simulink model "LinksMotorLinksAbbiegen"  (R2012b)
settings: Solver=ode45  StartTime=0.0  StopTime=11.0  RelTol=1e-3
undefined symbols (not defined in the file): sigbuilder_block
settings Model: Creator=mit064  LastModifiedBy=mit064

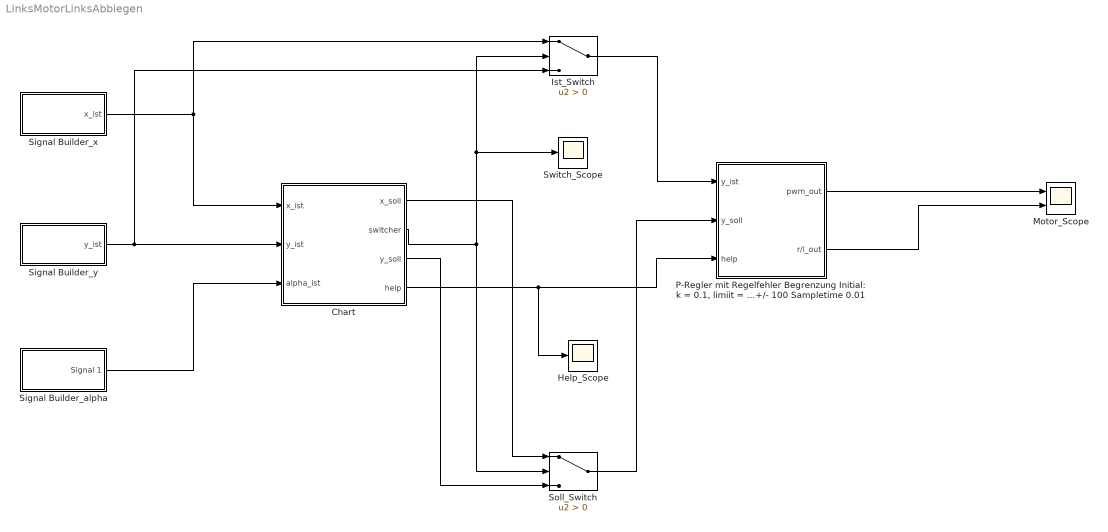
== system LinksMotorLinksAbbiegen ==
  Chart : Stateflow chart  TreatAsAtomicUnit=on
  Help_Scope : Scope
  Ist_Switch : Switch  Criteria=u2 > Threshold
  Motor_Scope : Scope  NumInputPorts=2
      settings: YMin=0~-5  YMax=100~5
  "P-Regler mit Regelfehler Begrenzung Initial: k = 0.1, limiit = +/- 100 Sampletime 0.01" : Subsystem
  Signal Builder_alpha : Subsystem  Tag=STV Subsys  LoadFcn=sigbuilder_block('load',[640.5 232.5 550.5 399.75 ]);  StartFcn=sigbuilder_block('start');  StopFcn=sigbuilder_block('stop');  ClipboardFcn=sigbuilder_block('clipboard');  mask(Sigbuilder block){}
      mask help: Simulink:masks:SigbuilderBlock_MD
      mask init:
      | if ~strcmp(get_param(bdroot(gcbh),'SimulationStatus'),'stopped') tuvar = sigbuilder_block('maskInit'); end
      settings: CopyFcn=sigbuilder_block('copy');  DeleteFcn=sigbuilder_block('delete');  ModelCloseFcn=sigbuilder_block('modelClose');  PreSaveFcn=sigbuilder_block('preSave');  PauseFcn=sigbuilder_block('pause');  ContinueFcn=sigbuilder_block('continue');  NameChangeFcn=sigbuilder_block('namechange');  OpenFcn=sigbuilder_block('open',[621.75 24.75 550.5 399.75 ]);  CloseFcn=sigbuilder_block('close');
      mask Display: plot(0, 0, 100, 100,[2, 2, 32, 32, 2], [68, 8, 8, 68, 68],[32, 2], [38, 38], [32, 19, 2],[53, 60, 44], [32, 17, 17, 2],[16, 16, 31, 31]);txt = getActiveGroup(gcbh);text(2, 100, txt,'verticalAlignment', 'top');
  Signal Builder_x : Subsystem  Tag=STV Subsys  LoadFcn=sigbuilder_block('load',[717.75 289.5 550.5 399.75 ]);  StartFcn=sigbuilder_block('start');  StopFcn=sigbuilder_block('stop');  ClipboardFcn=sigbuilder_block('clipboard');  mask(Sigbuilder block){}
      mask help: Simulink:masks:SigbuilderBlock_MD
      mask init:
      | if ~strcmp(get_param(bdroot(gcbh),'SimulationStatus'),'stopped') tuvar = sigbuilder_block('maskInit'); end
      settings: CopyFcn=sigbuilder_block('copy');  DeleteFcn=sigbuilder_block('delete');  ModelCloseFcn=sigbuilder_block('modelClose');  PreSaveFcn=sigbuilder_block('preSave');  PauseFcn=sigbuilder_block('pause');  ContinueFcn=sigbuilder_block('continue');  NameChangeFcn=sigbuilder_block('namechange');  OpenFcn=sigbuilder_block('open',[2.25 429.75 550.5 399.75 ]);  CloseFcn=sigbuilder_block('close');
      mask Display: plot(0, 0, 100, 100,[2, 2, 32, 32, 2], [68, 8, 8, 68, 68],[32, 2], [38, 38], [32, 19, 2],[53, 60, 44], [32, 17, 17, 2],[16, 16, 31, 31]);txt = getActiveGroup(gcbh);text(2, 100, txt,'verticalAlignment', 'top');
  Signal Builder_y : Subsystem  Tag=STV Subsys  LoadFcn=sigbuilder_block('load',[58.5 301.5 550.5 399.75 ]);  StartFcn=sigbuilder_block('start');  StopFcn=sigbuilder_block('stop');  ClipboardFcn=sigbuilder_block('clipboard');  mask(Sigbuilder block){}
      mask help: Simulink:masks:SigbuilderBlock_MD
      mask init:
      | if ~strcmp(get_param(bdroot(gcbh),'SimulationStatus'),'stopped') tuvar = sigbuilder_block('maskInit'); end
      settings: CopyFcn=sigbuilder_block('copy');  DeleteFcn=sigbuilder_block('delete');  ModelCloseFcn=sigbuilder_block('modelClose');  PreSaveFcn=sigbuilder_block('preSave');  PauseFcn=sigbuilder_block('pause');  ContinueFcn=sigbuilder_block('continue');  NameChangeFcn=sigbuilder_block('namechange');  OpenFcn=sigbuilder_block('open',[828.75 409.5 550.5 399.75 ]);  CloseFcn=sigbuilder_block('close');
      mask Display: plot(0, 0, 100, 100,[2, 2, 32, 32, 2], [68, 8, 8, 68, 68],[32, 2], [38, 38], [32, 19, 2],[53, 60, 44], [32, 17, 17, 2],[16, 16, 31, 31]);txt = getActiveGroup(gcbh);text(2, 100, txt,'verticalAlignment', 'top');
  Soll_Switch : Switch  Criteria=u2 > Threshold
  Switch_Scope : Scope
      settings: SaveName=ScopeData2
  wires:
  Chart/2(switcher) -> Soll_Switch/2, Switch_Scope/1, Ist_Switch/2
  Chart/1(x_soll) -> Soll_Switch/1
  Chart/3(y_soll) -> Soll_Switch/3
  Signal Builder_x/1(x_ist) -> Chart/1(x_ist), Ist_Switch/1
  Signal Builder_y/1(y_ist) -> Ist_Switch/3, Chart/2(y_ist)
  Signal Builder_alpha/1(Signal 1) -> Chart/3(alpha_ist)
  Ist_Switch/1 -> "P-Regler mit Regelfehler Begrenzung Initial: k = 0.1, limiit = +/- 100 Sampletime 0.01"/1(y_ist)
  Soll_Switch/1 -> "P-Regler mit Regelfehler Begrenzung Initial: k = 0.1, limiit = +/- 100 Sampletime 0.01"/2(y_soll)
  "P-Regler mit Regelfehler Begrenzung Initial: k = 0.1, limiit = +/- 100 Sampletime 0.01"/1(pwm_out) -> Motor_Scope/1
  "P-Regler mit Regelfehler Begrenzung Initial: k = 0.1, limiit = +/- 100 Sampletime 0.01"/2(r/l_out) -> Motor_Scope/2
  Chart/4(help) -> Help_Scope/1, "P-Regler mit Regelfehler Begrenzung Initial: k = 0.1, limiit = +/- 100 Sampletime 0.01"/3(help)

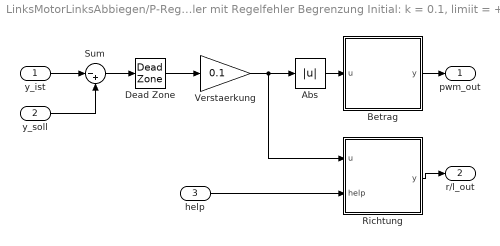
== system LinksMotorLinksAbbiegen/P-Regler mit Regelfehler Begrenzung Initial: k = 0.1, limiit = +//- 100 Sampletime 0.01 ==
  y_ist : Inport
  y_soll : Inport  Port=2
  help : Inport  Port=3
  Abs : Abs  SampleTime=0.01
  Betrag : MATLAB Function  TreatAsAtomicUnit=on  SystemSampleTime=0.01
  Dead Zone : DeadZone  LowerValue=-5  UpperValue=5  SampleTime=0.01  SaturateOnIntegerOverflow=on
  Richtung : MATLAB Function  TreatAsAtomicUnit=on  SystemSampleTime=0.01
  Sum : Sum  Inputs=|-+  SampleTime=0.01
  Verstaerkung : Gain  Gain=0.1  SampleTime=0.01
  pwm_out : Outport
  r/l_out : Outport  Port=2
  wires:
  Betrag/1(y) -> pwm_out/1
  Sum/1 -> Dead Zone/1
  Verstaerkung/1 -> Abs/1, Richtung/1(u)
  Dead Zone/1 -> Verstaerkung/1
  Abs/1 -> Betrag/1(u)
  y_soll/1 -> Sum/2
  Richtung/1(y) -> r/l_out/1
  y_ist/1 -> Sum/1
  help/1 -> Richtung/2(help)

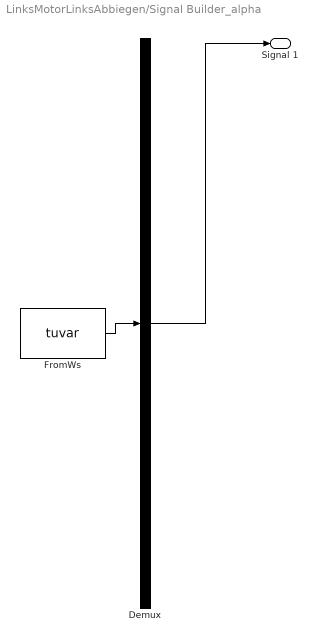
== system LinksMotorLinksAbbiegen/Signal Builder_alpha ==
  Demux : Demux  Tag=STV Demux  Outputs=1
  FromWs : FromWorkspace  Tag=STV FromWs  VariableName=tuvar  SampleTime=0
      SigBuilderData=|
      | common.afterFinalStr = 'Extrapolate'
      | common.sampleTime = 0
      | dataSet.timeRange = [0 11]
      | dataSet.name = 'Group 1'
      | sbobj.Groups.Name = 'Group 1'
      | sbobj.Groups.Signals.Name = 'Signal 1'
      | sbobj.Groups.Signals.XData = [0 5 7 11]
      | sbobj.Groups.Signals.YData = [-59 -59 63 63]
      | sbobj.Groups.TimeRange = [0 11]
  Signal 1 : Outport  Tag=STV Outport
  wires:
  Demux/1 -> Signal 1/1
  FromWs/1 -> Demux/1

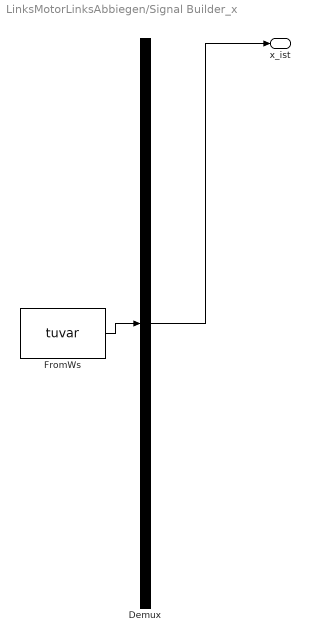
== system LinksMotorLinksAbbiegen/Signal Builder_x ==
  Demux : Demux  Tag=STV Demux  Outputs=1
  FromWs : FromWorkspace  Tag=STV FromWs  VariableName=tuvar  SampleTime=0
      SigBuilderData=|
      | common.afterFinalStr = 'Extrapolate'
      | common.sampleTime = 0
      | dataSet.timeRange = [0 11]
      | dataSet.name = 'Group 1'
      | sbobj.Groups.Name = 'Group 1'
      | sbobj.Groups.Signals.Name = 'x_ist'
      | sbobj.Groups.Signals.XData = [0 2 5 6.05 7.05 11]
      | sbobj.Groups.Signals.YData = [500 500 800 800 800 950]
      | sbobj.Groups.TimeRange = [0 11]
  x_ist : Outport  Tag=STV Outport
  wires:
  Demux/1 -> x_ist/1
  FromWs/1 -> Demux/1

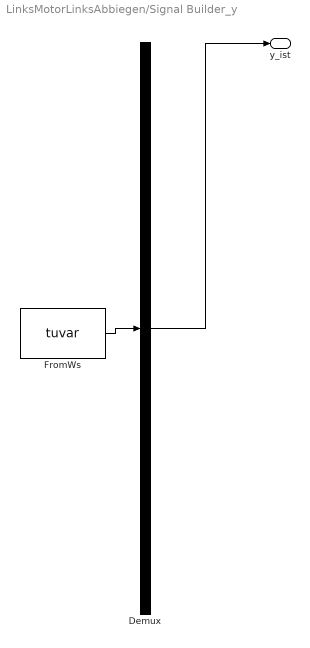
== system LinksMotorLinksAbbiegen/Signal Builder_y ==
  Demux : Demux  Tag=STV Demux  Outputs=1
  FromWs : FromWorkspace  Tag=STV FromWs  VariableName=tuvar  SampleTime=0
      SigBuilderData=|
      | common.afterFinalStr = 'Extrapolate'
      | common.sampleTime = 0
      | dataSet.timeRange = [0 11]
      | dataSet.name = 'Group 1'
      | sbobj.Groups.Name = 'Group 1'
      | sbobj.Groups.Signals.Name = 'y_ist'
      | sbobj.Groups.Signals.XData = [0 2 5 6 7 11]
      | sbobj.Groups.Signals.YData = [900 900 400 400 400 700]
      | sbobj.Groups.TimeRange = [0 11]
  y_ist : Outport  Tag=STV Outport
  wires:
  Demux/1 -> y_ist/1
  FromWs/1 -> Demux/1

== stateflow chart LinksMotorLinksAbbiegen/Chart ==
  state Start
  state Position_3
    switcher=0;
    help=1;
    state Position_2
      entry:y_soll=400;
    state Stop
      entry:y_soll=y_ist;
      exit:help=0;
    state Drehen_Linke
      entry:y_soll=0;
      exit:help=0;
    state stop
      entry:y_soll=y_ist;
      exit:help=0;
    state Position_4
      entry:y_soll=700
    (default) -> Position_2
    Position_2 -> Stop : [y_ist<402&&y_ist>398]
    Stop -> Drehen_Linke : [after(1,sec)]
    Drehen_Linke -> stop : [alpha_ist<65&&alpha_ist>61]
    stop -> Position_4 : [after(0.5,sec)]
  (default) -> Start
  Start -> Position_3 : [after(2,sec)]
  data: x_ist input; y_ist input; alpha_ist input; x_soll output; switcher output; y_soll output; help output

== matlab function LinksMotorLinksAbbiegen/P-Regler mit Regelfehler Begrenzung Initial: k = 0.1, limiit = +//- 100 Sampletime 0.01/Betrag ==
  settings: updateMethod=DISCRETE  sampleTime=0.01
  data: u input; y output
function y = fcn( u )

if 0.5 < u && u < 60
    y = 60;
elseif u <= 0.5
    y = 0;
elseif u >= 100
    y = 100;
else
    y = abs(u);
end

== matlab function LinksMotorLinksAbbiegen/P-Regler mit Regelfehler Begrenzung Initial: k = 0.1, limiit = +//- 100 Sampletime 0.01/Richtung ==
  settings: updateMethod=DISCRETE  sampleTime=0.01
  data: u input; y output; help input
function y = fcn( u,help )

if u > 0
    y = 1;
else
    y = 0+help;
end
